simulink model "ROSReady_FollowerStopper"  (R2019a)
settings: Solver=FixedStepAuto  StartTime=0.0  StopTime=800  FixedStep=0.01  RelTol=1e-3
settings Model: Creator=ckreienk  LastModifiedBy=ckreienk
settings DataIOCC: ReturnWorkspaceOutputs=off
settings DebuggingCC: ArithmeticOperatorsInVariantConditions=warning

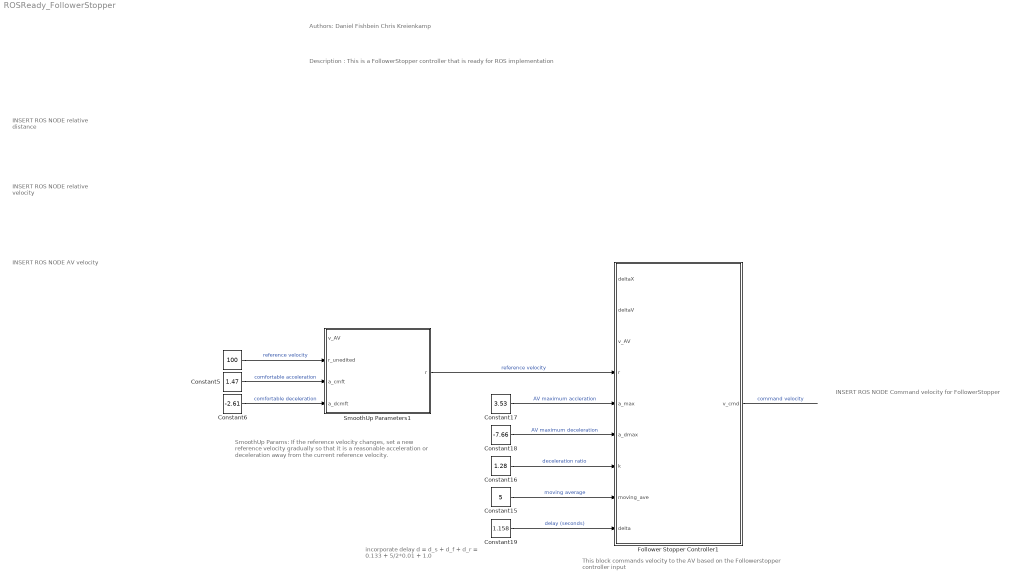
== system ROSReady_FollowerStopper ==
  note: Description : This is a FollowerStopper controller that is ready for ROS implementation
  note: Authors: Daniel Fishbein
      | Chris Kreienkamp
  note: INSERT ROS NODE
      | relative velocity
  note: INSERT ROS NODE
      | AV velocity
  note: INSERT ROS NODE
      | Command velocity for FollowerStopper
  note: INSERT ROS NODE
      | relative distance
  note: SmoothUp Params:
      | If the reference velocity changes,
      | set a new reference velocity gradually
      | so that it is a reasonable acceleration
      | or deceleration away from the current
      | reference velocity.
  note: This block commands velocity to the AV based
      | on the Followerstopper controller input
  note: incorporate delay
      | d = d_s + d_f + d_r
      | = 0.133 + 5/2*0.01 + 1.0
  "  " : Constant  Value=100
  Constant15 : Constant  Value=5
  Constant16 : Constant  Value=1.28
  Constant17 : Constant  Value=3.53
  Constant18 : Constant  Value=-7.66
  Constant19 : Constant  Value=1.158
  Constant5 : Constant  Value=1.47
  Constant6 : Constant  Value=-2.61
  Follower Stopper Controller1 : Subsystem
  SmoothUp Parameters1 : MATLAB Function  TreatAsAtomicUnit=on
  wires:
  ? -> Follower Stopper Controller1/1(deltaX)  "relative distance"
  ? -> Follower Stopper Controller1/2(deltaV)  "relative velocity"
  Constant6/1 -> SmoothUp Parameters1/4(a_dcmft)  "comfortable deceleration"
  Constant5/1 -> SmoothUp Parameters1/3(a_cmft)  "comfortable acceleration"
  ? -> Follower Stopper Controller1/3(v_AV), SmoothUp Parameters1/1(v_AV)  "AV velocity"
  "  "/1 -> SmoothUp Parameters1/2(r_unedited)  "reference velocity"
  Constant18/1 -> Follower Stopper Controller1/6(a_dmax)  "AV maximum deceleration"
  Constant19/1 -> Follower Stopper Controller1/9(delta)  "delay (seconds)"
  Constant17/1 -> Follower Stopper Controller1/5(a_max)  "AV maximum accleration"
  Constant15/1 -> Follower Stopper Controller1/8(moving_ave)  "moving average"
  Follower Stopper Controller1/1(v_cmd) -> ?  "command velocity"
  Constant16/1 -> Follower Stopper Controller1/7(k)  "deceleration ratio"
  SmoothUp Parameters1/1(r) -> Follower Stopper Controller1/4(r)  "reference velocity"

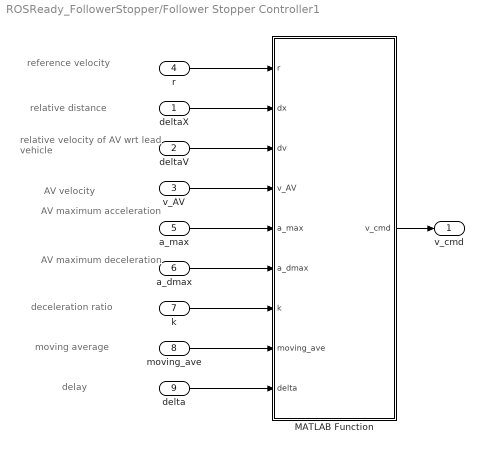
== system ROSReady_FollowerStopper/Follower Stopper Controller1 ==
  note: relative distance
  note: reference velocity
  note: AV velocity
  note: relative velocity of
      | AV wrt lead vehicle
  note: AV maximum
      | acceleration
  note: AV maximum
      | deceleration
  note: deceleration ratio
  note: moving average
  note: delay
  deltaX : Inport
  deltaV : Inport  Port=2
  v_AV : Inport  Port=3
  r : Inport  Port=4
  a_max : Inport  Port=5
  a_dmax : Inport  Port=6
  k : Inport  Port=7
  moving_ave : Inport  Port=8
  delta : Inport  Port=9
  MATLAB Function : MATLAB Function  TreatAsAtomicUnit=on
  v_cmd : Outport
  wires:
  r/1 -> MATLAB Function/1(r)
  v_AV/1 -> MATLAB Function/4(v_AV)
  MATLAB Function/1(v_cmd) -> v_cmd/1
  deltaV/1 -> MATLAB Function/3(dv)
  deltaX/1 -> MATLAB Function/2(dx)
  moving_ave/1 -> MATLAB Function/8(moving_ave)
  a_max/1 -> MATLAB Function/5(a_max)
  a_dmax/1 -> MATLAB Function/6(a_dmax)
  k/1 -> MATLAB Function/7(k)
  delta/1 -> MATLAB Function/9(delta)

== matlab function ROSReady_FollowerStopper/SmoothUp Parameters1 ==
  settings: updateMethod=DISCRETE
  data: v_AV input; r_unedited input; r output; a_cmft input; a_dcmft input
function r = fcn(v_AV,r_unedited,a_cmft,a_dcmft)
% #codegen
persistent y

if isempty(y)
    y=v_AV;
end

dt=0.01;
if( y > r_unedited + a_cmft*dt)
    y = max(r_unedited,y - abs(a_dcmft)*dt);
elseif( y < r_unedited - abs(a_dcmft)*dt)
    y = min(r_unedited,y + a_cmft*dt);
else
    y = r_unedited;
end

r = y;

== matlab function ROSReady_FollowerStopper/Follower Stopper Controller1/MATLAB Function ==
  settings: updateMethod=DISCRETE
  data: r input; dx input; dv input; v_cmd output; v_AV input; a_max input; a_dmax input; k input; moving_ave input; delta input
function v_cmd = fcn(r,dx,dv,v_AV,...
    a_max, a_dmax, k, moving_ave, delta)

%#codegen
% Safety controller, based on quadratic bands.
% Input: r = desired velocity (from other models)
%          dx = estimate of gap to vehicle ahead
%          dv = estimate of time derivative of dx (= velocity difference)
%        v_AV = velocity of AV
%      a_cmft = comfortable acceleration
%      a_dmax = maximum AV deceleration
%           k = ratio between maximum lead deceleration and a_dmax
%  moving_ave = number of v_cmd data points of which to take the average
% Out:  v_cmd = actual velocity commanded (always v_cmd<=r)
%
% Controller-specific parameters

% Lead vehicle velocity
v_lead = v_AV+dv; % velocity of lead vehicle
v_lead = max(v_lead,0); % lead vehicle cannot go backwards
v = min(r,v_lead); % safety velocity cannot exceed desired velocity r

% Relative distance parameters
deltaVSStar = max(1/(2*k*a_dmax)*(v_lead^2-k*v_AV^2),0);
dx1 = 1+deltaVSStar+v_AV*delta;
dx2 = dx1 + 2*v_AV*delta;
dx3 = 2*dx2-dx1;

% Actual commanded velocity
new_cmd = double((dx<=dx1).*(0))+...
    (dx1<dx&dx<=dx2).*(v*(dx-dx1)/(dx2-dx1))+...
    (dx2<dx&dx<=dx3).*(v + (r-v)*(dx-dx2)/(dx3-dx2))+...
    (dx3<dx).*(r);

% Take moving average of last moving_ave number of values
persistent moving_array
if isempty(moving_array)
    moving_array=zeros(1,moving_ave);
end
moving_array = [moving_array(2:moving_ave) new_cmd];
new_cmd_ave = mean(moving_array,'all');

% Make sure the moving average is within the maximum braking and maximum
% acceleration of the Ford Hybrid Escape
dt = 0.01;
possibleAcc = v_AV + a_max*dt;
possibleDec = v_AV + a_dmax*dt;
maxSafeSpeed = 27.24;
v_cmd = min(min(max(new_cmd_ave,possibleDec),possibleAcc), maxSafeSpeed);
